simulink model "aero421_finalProjectSim4_1"  (R2024a)
settings: Solver=FixedStepAuto  StartTime=0.0  StopTime=Period  FixedStep=10  RelTol=1e-3
values from neighbouring files (symbols this model uses):
  E0 = [phi0;theta0;psi0]    [aero421_finalProject.m]    (also in aero421_finalProject_D.m)
  q0 = [n0;e0]    [aero421_finalProject.m]    (also in aero421_finalProject_D.m)
  state_0 = [R_0';V_0']    [aero421_finalProject.m]    (also in aero421_finalProject_D.m)
undefined symbols (not defined in the file or in its folder): mehielSat
settings Model: Creator=emehiel  LastModifiedBy=tlunn
settings SolverCC: AlgebraicLoopSolver=TrustRegion
settings DebuggingCC: UnconnectedInputMsg=warning  UnconnectedOutputMsg=warning  UnconnectedLineMsg=warning
settings ModelReferenceCC: EnableRefExpFcnMdlSchedulingChecks=on
settings RTWCC: GPUComputeCapability=3.5

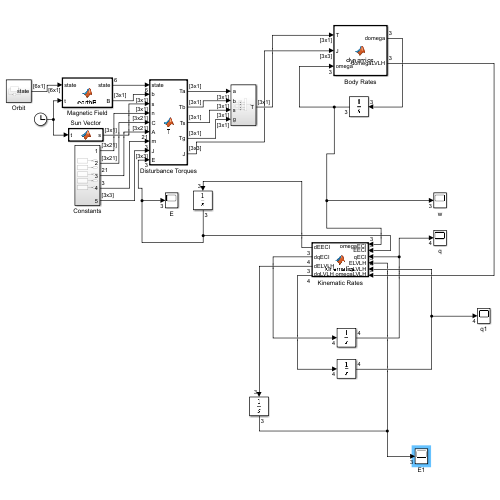
[thumbnail: Simulink's stored preview of the top-level diagram]
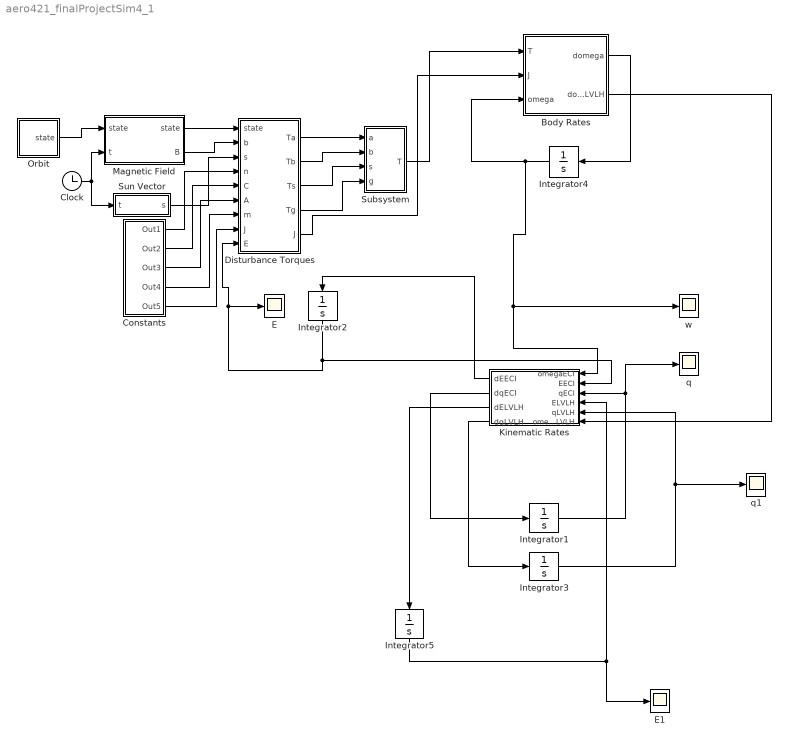
== system aero421_finalProjectSim4_1 ==
  Body Rates : MATLAB Function  TreatAsAtomicUnit=on
  Clock : Clock
  Constants : Subsystem
  Disturbance Torques : MATLAB Function  TreatAsAtomicUnit=on
  E : Scope
  E1 : Scope
  Integrator1 : Integrator  InitialCondition=q0
  Integrator2 : Integrator  InitialCondition=E0
  Integrator3 : Integrator  InitialCondition=q0
  Integrator4 : Integrator  InitialCondition=mehielSat.w0
  Integrator5 : Integrator  InitialCondition=E0
  Kinematic Rates : MATLAB Function  TreatAsAtomicUnit=on
  Magnetic Field : MATLAB Function  TreatAsAtomicUnit=on
  Orbit : Subsystem
  Subsystem : Subsystem
  Sun Vector : MATLAB Function  TreatAsAtomicUnit=on
  q : Scope
  q1 : Scope
  w : Scope
  wires:
  Body Rates/1(domega) -> Integrator4/1
  Integrator4/1 -> Body Rates/3(omega), Kinematic Rates/1(omegaECI), w/1
  Magnetic Field/2(B) -> Disturbance Torques/2(b)
  Sun Vector/1(s) -> Disturbance Torques/3(s)
  Constants/1(Out1) -> Disturbance Torques/4(n)
  Constants/2(Out2) -> Disturbance Torques/5(C)
  Constants/3(Out3) -> Disturbance Torques/6(A)
  Constants/4(Out4) -> Disturbance Torques/7(m)
  Constants/5(Out5) -> Disturbance Torques/8("J ")
  Kinematic Rates/1(dEECI) -> Integrator2/1
  Integrator2/1 -> E/1, Disturbance Torques/9(E), Kinematic Rates/2(EECI)
  Integrator1/1 -> Kinematic Rates/3(qECI), q/1
  Kinematic Rates/2(dqECI) -> Integrator1/1
  Orbit/1(state) -> Magnetic Field/1("state ")
  Clock/1 -> Magnetic Field/2(t), Sun Vector/1(t)
  Disturbance Torques/1(Ta) -> Subsystem/1(a)
  Disturbance Torques/2(Tb) -> Subsystem/2(b)
  Disturbance Torques/3(Ts) -> Subsystem/3(s)
  Disturbance Torques/4(Tg) -> Subsystem/4(g)
  Subsystem/1(T) -> Body Rates/1(T)
  Disturbance Torques/5(J) -> Body Rates/2(J)
  Magnetic Field/1(state) -> Disturbance Torques/1(state)
  Kinematic Rates/4(dqLVLH) -> Integrator3/1
  Integrator3/1 -> q1/1, Kinematic Rates/5(qLVLH)
  Kinematic Rates/3(dELVLH) -> Integrator5/1
  Integrator5/1 -> E1/1, Kinematic Rates/4(ELVLH)
  Body Rates/2(domegaLVLH) -> Kinematic Rates/6(omegaLVLH)

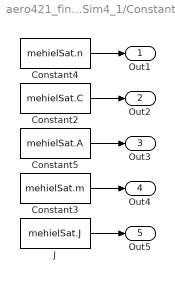
== system aero421_finalProjectSim4_1/Constants ==
  Constant2 : Constant  Value=mehielSat.C
  Constant3 : Constant  Value=mehielSat.m
  Constant4 : Constant  Value=mehielSat.n
  Constant5 : Constant  Value=mehielSat.A
  J : Constant  Value=mehielSat.J
  Out1 : Outport
  Out2 : Outport  Port=2
  Out3 : Outport  Port=3
  Out4 : Outport  Port=4
  Out5 : Outport  Port=5
  wires:
  J/1 -> Out5/1
  Constant2/1 -> Out2/1
  Constant3/1 -> Out4/1
  Constant4/1 -> Out1/1
  Constant5/1 -> Out3/1

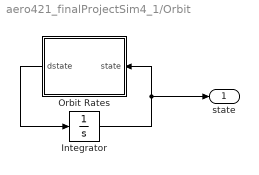
== system aero421_finalProjectSim4_1/Orbit ==
  Integrator : Integrator  InitialCondition=state_0
  Orbit Rates : MATLAB Function  TreatAsAtomicUnit=on
  state : Outport
  wires:
  Integrator/1 -> Orbit Rates/1(state), state/1
  Orbit Rates/1(dstate) -> Integrator/1

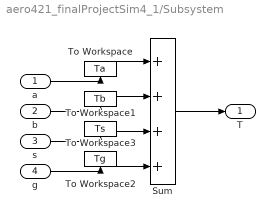
== system aero421_finalProjectSim4_1/Subsystem ==
  a : Inport
  b : Inport  Port=2
  s : Inport  Port=3
  g : Inport  Port=4
  Sum : Sum  Inputs=|++++
  To Workspace : ToWorkspace  VariableName=Ta  SampleTime=-1
  To Workspace1 : ToWorkspace  VariableName=Tb  SampleTime=-1
  To Workspace2 : ToWorkspace  VariableName=Tg  SampleTime=-1
  To Workspace3 : ToWorkspace  VariableName=Ts  SampleTime=-1
  T : Outport
  wires:
  s/1 -> To Workspace3/1, Sum/3
  b/1 -> To Workspace1/1, Sum/2
  Sum/1 -> T/1
  a/1 -> To Workspace/1, Sum/1
  g/1 -> To Workspace2/1, Sum/4

== matlab function aero421_finalProjectSim4_1/Magnetic Field ==
  data: state output; state input; t input; B output
function [state,B] = earthB(state,t)

i = t;

sec = rem(i,60);
i = (i - sec) / 60;

min = rem(i,60);
i = (i - min) / 60;

hrs = rem(i,24);
i = (i - hrs) / 24;

day = rem(i,31)+20;
i = (i - (day-1)) / 31;

mon = rem(i,12)+3;
i = (i - (mon-1)) / 12;

yrs = i + 2024;

time = [yrs mon day hrs min sec];

% initialize aerospace toolbox functions into simulink
coder.extrinsic("eci2ecef")
coder.extrinsic("ecef2eci")

% Initialize r vector in simulink for type setting
r = zeros(3,1);

% convert current r from eci to ecef
r = eci2ecef(time,state(1:3)); % km
r = r * 1000; % m
r_= norm(r);  % norm of r calculated for effeciency

a =   6371.2; % km
a = a * 1000; %  m

g11 = -1450.9;  % nT
h11 =  4652.5;  % nT
g01 =-29404.8;  % nT

g11 = g11 * 10^-9;  % T
h11 = h11 * 10^-9;  % T
g01 = g01 * 10^-9;  % T

m = a^3 * [g11;h11;g01]; % m^3*T

B = ((3 * m'*r) * r - r_^2 * m) / r_^5; % T
B = ecef2eci(time,B); % Convert B vector into ECI

end

== matlab function aero421_finalProjectSim4_1/Disturbance Torques ==
  data: state input; b input; s input; n input; C input; A input; m input; J input; Ta output; Tb output; Ts output; Tg output; E input; J output
function [Ta,Tb,Ts,Tg,J] = T(state,b,s,n,C,A,m,J,E)

% s,b,state input in ECI
% n,C,m,J input in Body
% A input in scalar

% T output needs to be in body

% Pull out R and V vectors from state vector
R = state(1:3);
V = state(4:6);

% Pull out Euler angles from E vector
phi   = E(1);
theta = E(2);
psi   = E(3);

% Use euler angles to calculate rotation matrix from ECI to body
C_ECI_B = basicrot(1,phi)*basicrot(2,theta)*basicrot(3,psi);

% Use rotation matrix to get ECI vectors into body
rb = C_ECI_B*R*1000; % R in meters
V  = C_ECI_B*V*1000; % V in m/s
s  = C_ECI_B*s;      % Sun direction vector
b  = C_ECI_B*b;      % Earth's magnetic field

%% Atmospheric Drag Torque, Ta

% Atmospherice Drag Torgue, preallocated
Ta = zeros(3,1);

% s/c velocity
v = norm(V); % speed, m/s
vhat = V/v; % velocity as unit vector, m/s 

% constants
rhoA = 1.644608e-14; % Atmospheric Density, kg/m^3
Cd = 2.5; % Coefficient of Drag, unitless

for i = 1:21
    if dot(n(:,i),vhat) > 0
        Cp = C(:,i); % center of pressure, m
        Fa = 1/2 * rhoA * v^2 * Cd * A(i) * vhat; % Drag Force, N
        Ta = Ta + cross(Cp,Fa); % Atmospheric Drag Torque, N*m
    end
end

%% Magnetic Field Torque, Tb
Tb = cross(m,b); % N*m

%% SRP Torque, Ts

% Preallocated SRP Torque Vector
Ts = zeros(3,1);

% constants 
p = 4.5e-6; % Solar Pressure in Earth Orbit, in N/m^2

for i = 1:21
    if dot(n(:,i),s) > 0
        Cp = C(:,i);
        Fa = -p * s * A(i); % SRP force on s/c, N
        Ts = Ts + cross(Cp,Fa); % SRP Torque, N*m
    end
end

%% Gravity Gradient Torque, Tg

% constants
mu = 3.98600e14; % gravitational parameter kg^2/m^3

rx = vect2cross(rb); % vector cross of position vector, m

Tg = ((3 * mu) / norm(rb)^5) * rx * J * rb; % Gravity Gradient Torque, N*m

%% Sub Functions
function ax = vect2cross(a)

ax = [0 -a(3) a(2); a(3) 0 -a(1); -a(2) a(1) 0];

end

function [C] = basicrot(a,theta)

if a == 1
    C = [1 0 0 ; 0 cosd(theta) sind(theta); 0 -sind(theta) cosd(theta)];
elseif a == 2
    C = [cosd(theta) 0 -sind(theta); 0 1 0; sind(theta) 0 cosd(theta)];
elseif a == 3
    C = [cosd(theta) sind(theta) 0; -sind(theta) cosd(theta) 0; 0 0 1];
end
end


end

== matlab function aero421_finalProjectSim4_1/Orbit/Orbit Rates ==
  data: dstate output; state input
function dstate  = orbitRates(state)

mu = 398600; % gravitational parameter, in km

x = state(1);
y = state(2);
z = state(3);
dx = state(4);
dy = state(5);
dz = state(6);

r = norm([x y z]);

ddx = -mu * x / r^3;
ddy = -mu * y / r^3;
ddz = -mu * z / r^3;

dstate = [dx;dy;dz;ddx;ddy;ddz];

== matlab function aero421_finalProjectSim4_1/Body Rates ==
  data: T input; J input; omega input; domega output; domegaLVLH output
function [domega,domegaLVLH] = dynamics(T, J, omega)
%#codegen

% Compute the derivative of the angular velocity $\omega$ here

% Using the Euler Equations

wXdot_ECI = (T(1)-(J(3,3)-J(2,2))*omega(2)*omega(3))/J(1,1);
wYdot_ECI = (T(2)-(J(1,1)-J(3,3))*omega(1)*omega(3))/J(2,2);
wZdot_ECI = (T(3)-(J(2,2)-J(1,1))*omega(1)*omega(2))/J(3,3);
domega = [wXdot_ECI; wYdot_ECI; wZdot_ECI];

Period = 5.999942157180395e+03;

omegaLVLH_ECI = [0;((2*pi)/Period);0];

omegaLVLH = omega-omegaLVLH_ECI;

wXdot_LVLH = (T(1)-(J(3,3)-J(2,2))*omegaLVLH(2)*omegaLVLH(3))/J(1,1);
wYdot_LVLH = (T(2)-(J(1,1)-J(3,3))*omegaLVLH(1)*omegaLVLH(3))/J(2,2);
wZdot_LVLH = (T(3)-(J(2,2)-J(1,1))*omegaLVLH(1)*omegaLVLH(2))/J(3,3);
domegaLVLH = [wXdot_LVLH; wYdot_LVLH; wZdot_LVLH];

== matlab function aero421_finalProjectSim4_1/Sun Vector ==
  data: t input; s output
function s = sunVector(t)

% https://www.mathworks.com/matlabcentral/fileexchange/114710-investigation-of-the-sun-direction-vector-in-eci

JD = 2.4603895e+06 + (t/86400);

T_UT1= (JD - 2451545)/36525;
% The mean longitude of the sun
delta_M_Sun= 280.460 + 36000.770*T_UT1;
T_TDB= T_UT1;
% The mean anomaly of the sun
M_Sun= 357.5277233 + 35999.05034*T_TDB;
% The ecliptic longitude of the sun
delta_ecliptic= delta_M_Sun + 1.914666471*sind(M_Sun) + 0.019994643*sin(2*M_Sun);
% The linear model of the ecliptic of the sun
E= 23.439291 - 0.0130042*T_TDB;
% The unit sun vector is given in the ECI frame
s = [cosd(delta_ecliptic); sind(delta_ecliptic).*cosd(E); sind(delta_ecliptic).*sind(E)];

== matlab function aero421_finalProjectSim4_1/Kinematic Rates ==
  data: dEECI output; dqECI output; dELVLH output; omegaECI input; EECI input; qECI input; dqLVLH output; ELVLH input; qLVLH input; omegaLVLH input
function [dEECI,dqECI,dELVLH,dqLVLH] = kinematics(omegaECI,EECI,qECI,ELVLH,qLVLH,omegaLVLH)
%#codegen

% unpack quaternion

% compute the derivative of the quaternion components here

% compute the derivative of the Euler Angle components here


% The spacecraft initial attitude is such that it is aligned with F_LVLH
% Compute initial quaternion and EULER angles relating Fb and Feci

nECI = qECI(1);
eECI = qECI(2:4);

% Rates In ECI

dnECI =-1/2 * eECI' * omegaECI;
deECI = 1/2 * (nECI * eye(3) + vect2cross(eECI)) * omegaECI;

dqECI = [dnECI; deECI];

phiECI   = EECI(1);
thetaECI = EECI(2);

dEECI = [1, sin(phiECI)*tan(thetaECI), cos(phiECI)*tan(thetaECI); ...
     0, cos(phiECI)           ,-sin(phiECI);            ...
     0, sin(phiECI)*sec(thetaECI), cos(phiECI)*sec(thetaECI)] * omegaECI;

% Rates In LVLH

nLVLH = qLVLH(1);
eLVLH = qLVLH(2:4);

dnLVLH = -1/2 * eLVLH' * omegaLVLH;
deLVLH = 1/2 * (nLVLH * eye(3) + vect2cross(eLVLH)) * omegaLVLH;

dqLVLH = [dnLVLH; deLVLH];

phiLVLH   = ELVLH(1);
thetaLVLH = ELVLH(2);

dELVLH = [1, sin(phiLVLH)*tan(thetaLVLH), cos(phiLVLH)*tan(thetaLVLH); ...
     0, cos(phiLVLH)           ,-sin(phiLVLH);            ...
     0, sin(phiLVLH)*sec(thetaLVLH), cos(phiLVLH)*sec(thetaLVLH)] * omegaLVLH;

function ax = vect2cross(a)

ax = [0 -a(3) a(2); a(3) 0 -a(1); -a(2) a(1) 0];

end

end
